simulink model "exampleTask"  (R2018a)
settings: Solver=VariableStepAuto  StartTime=0.0  StopTime=100  RelTol=1e-3
settings Model: Creator=fignigno  LastModifiedBy=fignigno

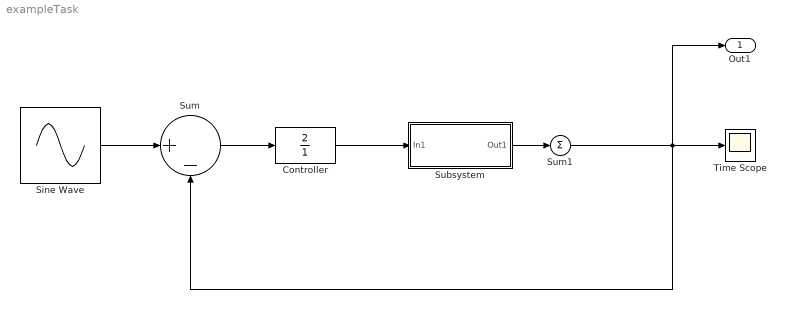
== system exampleTask ==
  Controller : TransferFcn  Numerator=[2]  Denominator=[1]
  Sine Wave : Sin  SampleTime=0
  Subsystem : Subsystem
  Sum : Sum  Inputs=|+-
  Sum1 : Sum  Inputs=+
  Time Scope : Scope
  Out1 : Outport
  wires:
  Sum/1 -> Controller/1
  Sine Wave/1 -> Sum/1
  Sum1/1 -> Out1/1, Time Scope/1, Sum/2
  Controller/1 -> Subsystem/1(In1)
  Subsystem/1(Out1) -> Sum1/1

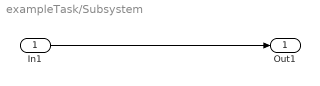
== system exampleTask/Subsystem ==
  In1 : Inport
  Out1 : Outport
  wires:
  In1/1 -> Out1/1
